simulink subsystem "Day2_Scenario_2_3"  (R2024a)
settings: Solver=VariableStepAuto  StartTime=0.0  StopTime=10.0  RelTol=1e-3
libraries: CarMaker4SL x6
settings Model: Creator=junhyung.cha  LastModifiedBy=User

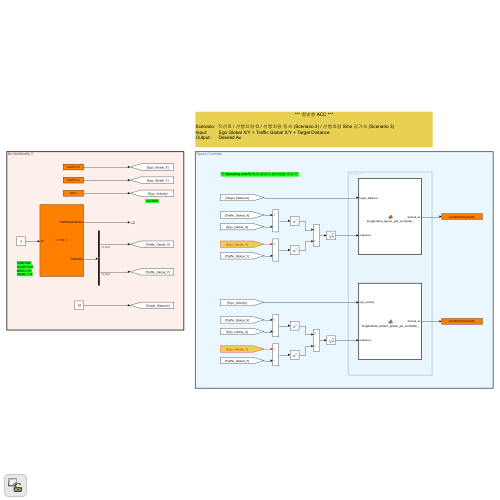
[thumbnail: Simulink's stored preview of the top-level diagram]
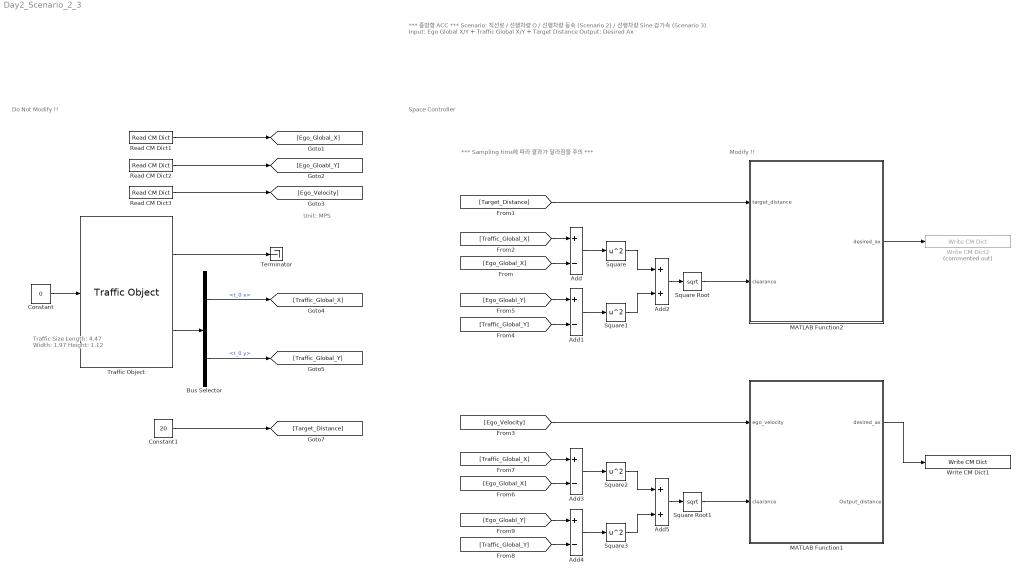
== system Day2_Scenario_2_3 ==
  note: *** Sampling time에 따라 결과가 달라짐을 주의 ***
  note: Space Controller
  note: Modify !!
  note: Do Not Modify !!
  note: Traffic Size
      | Length: 4.47
      | Width: 1.97
      | Height: 1.12
  note: *** 종방향 ACC ***
      |
      | Scenario: 직선로 / 선행차량 O / 선행차량 등속 (Scenario 2) / 선행차량 Sine 감가속 (Scenario 3)
      | Input: Ego Global X/Y + Traffic Global X/Y + Target Distance
      | Output: Desired Ax
  note: Unit: MPS
  Add{,1,3..4} (4 alike) : Sum  Inputs=+-
  Add2 : Sum
  Add5 : Sum
  Bus Selector : BusSelector  OutputSignals=t_0 x,t_0 y
  Constant : Constant  Value=0
  Constant1 : Constant  Value=20
  MATLAB Function1 : MATLAB Function  TreatAsAtomicUnit=on
  MATLAB Function2 : MATLAB Function  TreatAsAtomicUnit=on
  Read CM Dict1 : CarMaker4SL/Read CM Dict  xname=Car.Fr1.tx  xsync=off  xstime=Inherited
  Read CM Dict2 : CarMaker4SL/Read CM Dict  xname=Car.Fr1.ty  xsync=off  xstime=Inherited
  Read CM Dict3 : CarMaker4SL/Read CM Dict  xname=Car.v  xsync=off  xstime=Inherited
  Square{,1..3} (4 alike) : Math  Operator=square
  Square Root : Sqrt
  Square Root1 : Sqrt
  Terminator : Terminator
  Traffic Object : CarMaker4SL/Traffic Object  xname=T00  ximode=Traffic Id  xstime=Inherited
      settings: SourceProductName=CarMaker4SL
  Write CM Dict1 : CarMaker4SL/Write CM Dict  xname=AccelCtrl.DesiredAx  xsync=off
  Write CM Dict2 : CarMaker4SL/Write CM Dict  Commented=on  xname=AccelCtrl.DesiredAx  xsync=off
  wires:
  Read CM Dict2/1 -> [Ego_Gloabl_Y]
  MATLAB Function2/1(desired_ax) -> Write CM Dict2/1
  Read CM Dict1/1 -> [Ego_Global_X]
  Constant/1 -> Traffic Object/1
  Traffic Object/2 -> Bus Selector/1
  Traffic Object/1 -> Terminator/1
  Bus Selector/1 -> [Traffic_Global_X]  "<t_0 x>"
  Bus Selector/2 -> [Traffic_Global_Y]  "<t_0 y>"
  Square Root/1 -> MATLAB Function2/2(clearance)
  Constant1/1 -> [Target_Distance]
  [Ego_Global_X] -> Add/2
  [Traffic_Global_X] -> Add/1
  [Traffic_Global_Y] -> Add1/2
  [Ego_Gloabl_Y] -> Add1/1
  Add1/1 -> Square1/1
  Add2/1 -> Square Root/1
  Square/1 -> Add2/1
  Square1/1 -> Add2/2
  [Target_Distance] -> MATLAB Function2/1(target_distance)
  Add/1 -> Square/1
  Read CM Dict3/1 -> [Ego_Velocity]
  [Ego_Velocity] -> MATLAB Function1/1(ego_velocity)
  Add3/1 -> Square2/1
  Square3/1 -> Add5/2
  Square2/1 -> Add5/1
  Add5/1 -> Square Root1/1
  Add4/1 -> Square3/1
  [Ego_Gloabl_Y] -> Add4/1
  [Traffic_Global_Y] -> Add4/2
  [Traffic_Global_X] -> Add3/1
  [Ego_Global_X] -> Add3/2
  Square Root1/1 -> MATLAB Function1/2(clearance)
  MATLAB Function1/1(desired_ax) -> Write CM Dict1/1

== matlab function Day2_Scenario_2_3/MATLAB Function2 ==
  settings: updateMethod=DISCRETE  sampleTime=0.05
  data: target_distance input; desired_ax output; clearance input
function desired_ax = longitudinal_space_pid_controller_(target_distance, clearance)
    %#codegen
    
    % PID Controller parameters
    persistent integral prev_error; % Persistent variables to store integral and previous error
    Kp = 0.4; % Proportional gain
    Ki = 0.07; % Integral gain
    Kd = 0.25; % Derivative gain
    step_time = 0.01; % Fixed time interval for sampling (update as needed)
    
    if isempty(integral)
        integral = 0;      % Initialize integral during the first step
        prev_error = 0;     % Initialize previous error
    end
    
    % Error calculation
    error = clearance - target_distance;
    
    % Proportional term
    P_term = Kp * error;
    
    % Integral term
    integral = integral + error * step_time;
    I_term = Ki * integral;
    
    % Derivative term
    derivative = (error - prev_error) / step_time;
    D_term = Kd * derivative;
    
    % PID control output (desired acceleration)
    desired_ax = P_term + I_term + D_term;
    
    % Update previous error
    prev_error = error;

end

== matlab function Day2_Scenario_2_3/MATLAB Function1 ==
  settings: updateMethod=DISCRETE  sampleTime=0.05
  data: ego_velocity input; desired_ax output; clearance input; Output_distance output
function [desired_ax,Output_distance] = longitudinal_variant_space_pd_controller_(ego_velocity, clearance)
    persistent prev_error initialized

    dt = 0.001;

    % 거리 기반 PID 제어 (PD 버전)
    Kp = 0.8;
    Kd = 0.4;

    % 시간 간격 기반 목표 거리 설정
    d0 = 5;      % 최소 안전 거리 (m)
    time_gap = 1.5;  % 시간 간격 (s)
    Output_distance = d0 + time_gap * ego_velocity;

    if isempty(initialized)
        prev_error = 0;
        initialized = true;
    end

    % 거리 기반 오차 및 미분
    error = Output_distance - clearance;
    derivative = (error - prev_error) / dt;

    
    % 거리 기반 제어기 출력
    desired_ax = - (Kp * error + Kd * derivative);

    % 상태 업데이트
    prev_error = error;
end
